simulink subsystem "mean_with_reset"  (R2020b)
settings: Solver=VariableStepAuto  StartTime=0.0  StopTime=10.0  RelTol=1e-3
settings Model: Creator=Utente CAL  LastModifiedBy=Previ

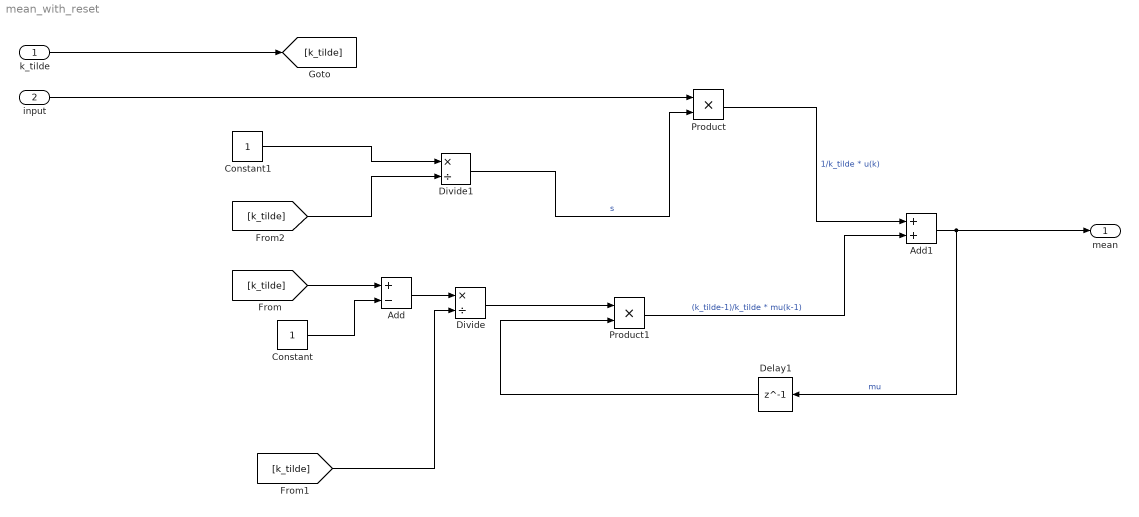
== system mean_with_reset ==
  k_tilde : Inport
  input : Inport  Port=2
  Add : Sum  Inputs=+-  RndMeth=Nearest
  Add1 : Sum  OutDataTypeStr=double  RndMeth=Nearest
  Constant : Constant
  Constant1 : Constant
  Delay1 : Delay  DelayLength=1  InitialCondition=0  SampleTime=1
  Divide : Product  Inputs=*/  RndMeth=Nearest
  Divide1 : Product  Inputs=*/  InputSameDT=on  RndMeth=Nearest
  Product : Product  RndMeth=Nearest
  Product1 : Product  RndMeth=Nearest
  mean : Outport
  wires:
  Divide/1 -> Product1/1
  Constant/1 -> Add/2
  [k_tilde] -> Divide/2
  [k_tilde] -> Add/1
  Constant1/1 -> Divide1/1
  Product1/1 -> Add1/2  "(k_tilde-1)/k_tilde * mu(k-1)"
  [k_tilde] -> Divide1/2
  Add/1 -> Divide/1
  Product/1 -> Add1/1  "1/k_tilde * u(k)"
  Add1/1 -> mean/1, Delay1/1  "mu"
  input/1 -> Product/1
  k_tilde/1 -> [k_tilde]
  Delay1/1 -> Product1/2
  Divide1/1 -> Product/2  "s"
